simulink model "ysw9_1sim"  (R2014a)
settings: Solver=ode45  StartTime=0.0  StopTime=30  RelTol=1e-3
settings Model: ExtModeTrigMode=oneshot  ExtModeArmWhenConnect=off  Creator=ljk  LastModifiedBy=ii
settings DataIOCC: Decimation=100  LimitDataPoints=off  SignalLoggingSaveFormat=ModelDataLogs  SaveOutput=off  SaveTime=off  SignalLoggingName=sigsOut
settings OptimizationCC: BooleanDataType=off  ExpressionDepthLimit=2147483647
settings DebuggingCC: SaveWithParameterizedLinksMsg=none  UnderspecifiedInitializationDetection=Classic  SignalResolutionControl=TryResolveAllWithWarning  SolverPrmCheckMsg=none  MultiTaskDSMMsg=warning  MultiTaskCondExecSysMsg=none  FcnCallInpInsideContextMsg=UseLocalSettings  StateNameClashWarn=warning
settings HardwareCC: TargetUnknown=on
settings RTWCC: IncludeERTFirstTime=on
settings GRTTargetCC: CombineOutputUpdateFcns=off  GRTInterface=on

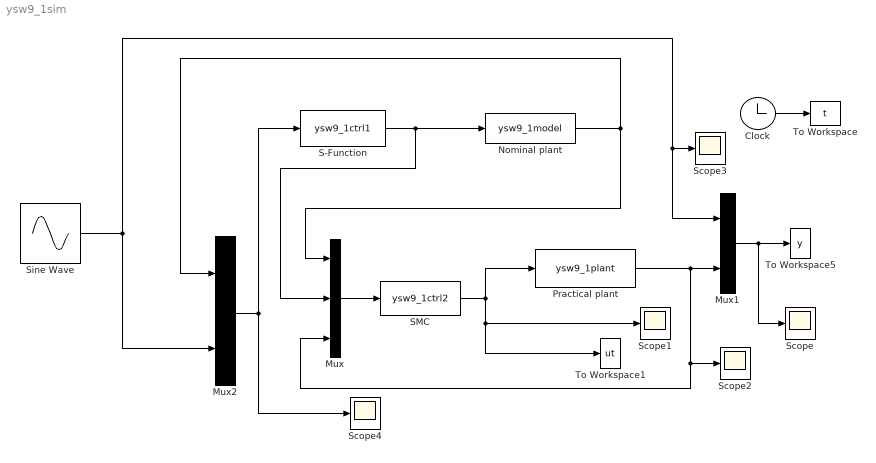
== system ysw9_1sim ==
  Clock : Clock
  Mux : Mux  Inputs=3
  Mux1 : Mux  Inputs=2
  Mux2 : Mux  Inputs=2
  Nominal plant : S-Function  FunctionName=ysw9_1model  EnableBusSupport=off
  Practical plant : S-Function  FunctionName=ysw9_1plant  EnableBusSupport=off
  S-Function : S-Function  FunctionName=ysw9_1ctrl1  EnableBusSupport=off
  SMC : S-Function  FunctionName=ysw9_1ctrl2  EnableBusSupport=off
  Scope{,1..4} (5 alike) : Scope
      Scope2 settings: SaveName=ScopeData2
      Scope3 settings: SaveName=ScopeData3
      Scope4 settings: SaveName=ScopeData4
  Sine Wave : Sin  SampleTime=0
  To Workspace : ToWorkspace  VariableName=t  SampleTime=-1
  To Workspace1 : ToWorkspace  VariableName=ut  SampleTime=-1
  To Workspace5 : ToWorkspace  VariableName=y  SampleTime=-1
  wires:
  Clock/1 -> To Workspace/1
  Mux/1 -> SMC/1
  SMC/1 -> Scope1/1, To Workspace1/1, Practical plant/1
  Mux2/1 -> Scope4/1, S-Function/1
  Mux1/1 -> Scope/1, To Workspace5/1
  Practical plant/1 -> Scope2/1, Mux/3, Mux1/2
  Nominal plant/1 -> Mux2/1, Mux/1
  S-Function/1 -> Nominal plant/1, Mux/2
  Sine Wave/1 -> Scope3/1, Mux1/1, Mux2/2
